simulink model "g_closed_loop_simulation"  (R2025a)
settings: Solver=VariableStepAuto  StartTime=0.0  StopTime=1.5  RelTol=1e-3
values from neighbouring files (symbols this model uses):
  B = 0    [Simulink_support_script.m]    (also in quick_pole_check.m)
  Jm = 5.508e-5    (= 5.508e-05)    [Simulink_support_script.m]
  K = 0.0991    [HW2_pro1_min_ab_plot_script.m]    (also in Simulink_support_script.m; quick_pole_check.m)
  L = 2.38e-3    (= 0.00238)    [Simulink_support_script.m]    (also in quick_pole_check.m = max(xr, yr))
  R = 1.43    [Simulink_support_script.m]    (also in quick_pole_check.m)
  stim_step = 100    [Simulink_support_script.m]
  Tl_final = 0.5    [Simulink_support_script.m]
  Tl_initial = 0    [Simulink_support_script.m]
  Tl_step_t = 0.05    [Simulink_support_script.m]
settings Model: Creator=lpurd  LastModifiedBy=lpurd

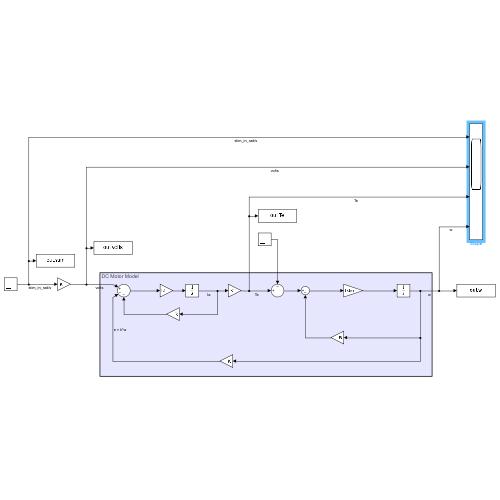
[thumbnail: Simulink's stored preview of the top-level diagram]
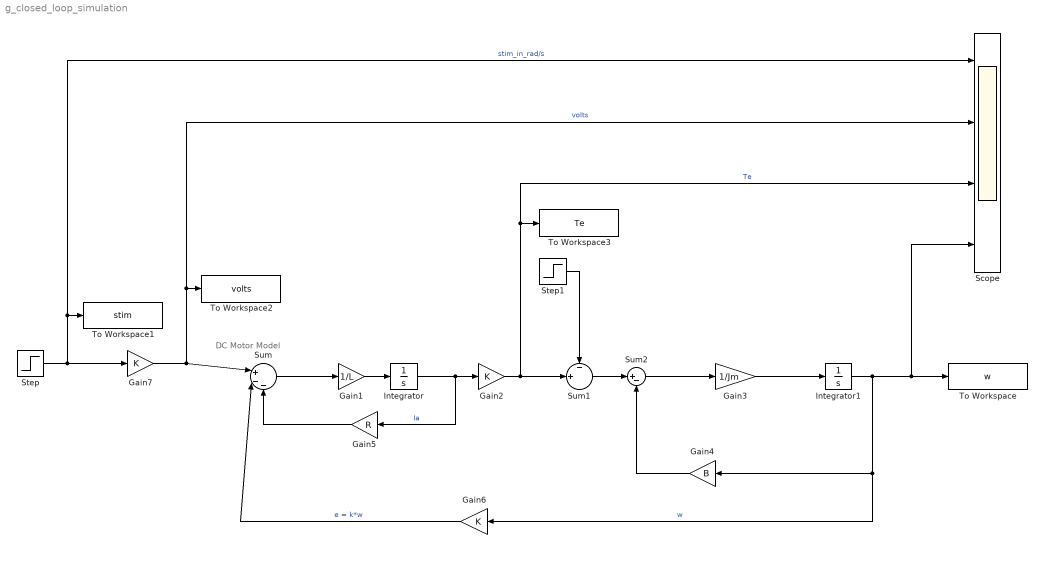
== system g_closed_loop_simulation ==
  note: DC Motor Model
  Gain1 : Gain  Gain=1/L
  Gain2 : Gain  Gain=K
  Gain3 : Gain  Gain=1/Jm
  Gain4 : Gain  Gain=B
  Gain5 : Gain  Gain=R
  Gain6 : Gain  Gain=K
  Gain7 : Gain  Gain=K
  Integrator : Integrator
  Integrator1 : Integrator
  Scope : Scope  NumInputPorts=4
      settings: ActiveDisplayYMinimum=-21.276316992913749  ActiveDisplayYMaximum=191.48685293622378
  Step : Step  Time=0  After=stim_step  SampleTime=0
  Step1 : Step  Time=Tl_step_t  Before=Tl_initial  After=Tl_final  SampleTime=0
  Sum : Sum  Inputs=|+--
  Sum1 : Sum  Inputs=-|+||
  Sum2 : Sum  Inputs=|+-
  To Workspace : ToWorkspace  VariableName=w  SaveFormat=Timeseries  SampleTime=-1
  To Workspace1 : ToWorkspace  VariableName=stim  SaveFormat=Timeseries  SampleTime=-1
  To Workspace2 : ToWorkspace  VariableName=volts  SaveFormat=Timeseries  SampleTime=-1
  To Workspace3 : ToWorkspace  VariableName=Te  SaveFormat=Timeseries  SampleTime=-1
  wires:
  Gain6/1 -> Sum/2  "e = k*w"
  Gain4/1 -> Sum2/2
  Gain5/1 -> Sum/3
  Gain2/1 -> Scope/3, To Workspace3/1, Sum1/2  "Te"
  Sum1/1 -> Sum2/1
  Sum2/1 -> Gain3/1
  Step1/1 -> Sum1/1
  Gain3/1 -> Integrator1/1
  Integrator1/1 -> Scope/4, To Workspace/1, Gain6/1, Gain4/1  "w"
  Sum/1 -> Gain1/1
  Gain1/1 -> Integrator/1
  Integrator/1 -> Gain5/1, Gain2/1  "Ia"
  Step/1 -> Scope/1, To Workspace1/1, Gain7/1  "stim_in_rad/s"
  Gain7/1 -> Scope/2, To Workspace2/1, Sum/1  "volts"
